simulink model "Breach_monitoring_subsystem"  (R2019b)
settings: Solver=VariableStepAuto  StartTime=0.0  StopTime=11.0  RelTol=1e-3
undefined symbols (not defined in the file or in its folder): nb_rooms, nb_step_to_fifteen_min, nb_step_to_one_h, nb_step_to_thirty_min
libraries: slstlib x6, dspstat3 x6
settings Model: Creator=pat  LastModifiedBy=pat

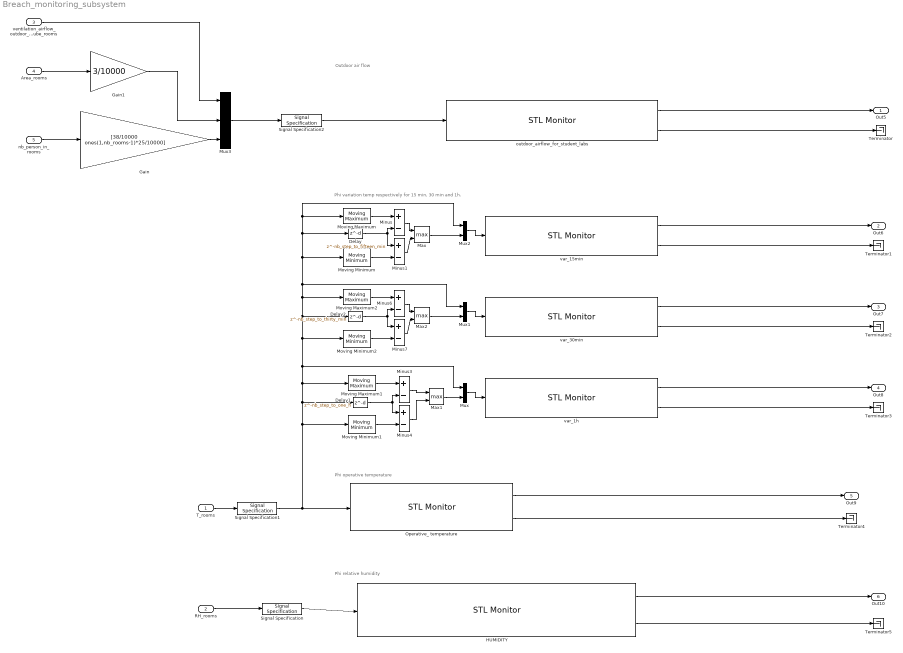
== system Breach_monitoring_subsystem ==
  note: Outdoor air flow
  note: Phi relative humidity
  note: Phi variation temp respectively for 15 min, 30 min and 1h.
  note: Phi operative temperature
  T_rooms : Inport  PortDimensions=nb_rooms
  RH_rooms : Inport  Port=2  PortDimensions=nb_rooms
  ventilation_airflow_outdoor_air_mcube_rooms : Inport  Port=3  PortDimensions=nb_rooms
  Area_rooms : Inport  Port=4  PortDimensions=nb_rooms
  nb_person_in_rooms : Inport  Port=5  OutDataTypeStr=double  PortDimensions=nb_rooms
  Delay : Delay  DelayLength=nb_step_to_fifteen_min  InitialCondition=0
  Delay1 : Delay  DelayLength=nb_step_to_one_h  InitialCondition=0
  Delay2 : Delay  DelayLength=nb_step_to_thirty_min  InitialCondition=0
  Gain : Gain  Gain=[38/10000 ones(1,nb_rooms-1)*25/10000]
  Gain1 : Gain  Gain=3/10000
  "HUMIDITY " : slstlib/STL Monitor  SignalNames=name_rh  STLString=formula_rh  MaxRob=1  RefreshRate=rate  rob_low_lim=inf  rob_up_lim=-inf  rob_diff_lim=-inf
      settings: SourceProductName=Breach Library
  Max : MinMax  Function=max  Inputs=2
  Max1 : MinMax  Function=max  Inputs=2
  Max2 : MinMax  Function=max  Inputs=2
  Minus{,1,3..4,6..7} (6 alike) : Sum  Inputs=+-
  Moving Maximum : dspstat3/Moving Maximum  SpecifyWindowLength=on  WindowLength=nb_step_to_fifteen_min  SimulateUsing=Code generation
      settings: SourceProductName=DSP System Toolbox  SourceProductBaseCode=DS
  Moving Maximum1 : dspstat3/Moving Maximum  SpecifyWindowLength=on  WindowLength=nb_step_to_one_h  SimulateUsing=Code generation
      settings: SourceProductName=DSP System Toolbox  SourceProductBaseCode=DS
  Moving Maximum2 : dspstat3/Moving Maximum  SpecifyWindowLength=on  WindowLength=nb_step_to_thirty_min  SimulateUsing=Code generation
      settings: SourceProductName=DSP System Toolbox  SourceProductBaseCode=DS
  Moving Minimum : dspstat3/Moving Minimum  SpecifyWindowLength=on  WindowLength=nb_step_to_fifteen_min  SimulateUsing=Code generation
      settings: SourceProductName=DSP System Toolbox  SourceProductBaseCode=DS
  Moving Minimum1 : dspstat3/Moving Minimum  SpecifyWindowLength=on  WindowLength=nb_step_to_one_h  SimulateUsing=Code generation
      settings: SourceProductName=DSP System Toolbox  SourceProductBaseCode=DS
  Moving Minimum2 : dspstat3/Moving Minimum  SpecifyWindowLength=on  WindowLength=nb_step_to_thirty_min  SimulateUsing=Code generation
      settings: SourceProductName=DSP System Toolbox  SourceProductBaseCode=DS
  Mux : Mux  Inputs=2
  Mux1 : Mux  Inputs=2
  Mux2 : Mux  Inputs=2
  Mux3 : Mux  Inputs=[nb_rooms nb_rooms nb_rooms]
  Operative_ temperature : slstlib/STL Monitor  SignalNames=name_op_temp  STLString=formula_op_temp  MaxRob=40  RefreshRate=rate  rob_low_lim=inf  rob_up_lim=-inf  rob_diff_lim=-inf
      settings: SourceProductName=Breach Library
  Signal Specification : SignalSpecification  OutMin=-0.25  OutMax=1.25  Dimensions=nb_rooms
  Signal Specification1 : SignalSpecification  OutMin=-100  OutMax=100  Dimensions=nb_rooms
  Signal Specification2 : SignalSpecification  OutMin=-10000  OutMax=10000  Dimensions=nb_rooms*3
  Terminator{,1..5} (6 alike) : Terminator
  outdoor_airflow_for_student_labs : slstlib/STL Monitor  SignalNames=name_out_airflow  STLString=formula_out_airflow  MaxRob=40  RefreshRate=rate  rob_low_lim=inf  rob_up_lim=-inf  rob_diff_lim=-inf
      settings: SourceProductName=Breach Library
  var_15min : slstlib/STL Monitor  SignalNames=name_variation  STLString=formula_fifteen_min_var  MaxRob=2  RefreshRate=rate  rob_low_lim=inf  rob_up_lim=-inf  rob_diff_lim=-inf
      settings: SourceProductName=Breach Library
  var_1h : slstlib/STL Monitor  SignalNames=name_variation  STLString=formula_one_h_var  MaxRob=2  RefreshRate=rate  rob_low_lim=inf  rob_up_lim=-inf  rob_diff_lim=-inf
      settings: SourceProductName=Breach Library
  var_30min : slstlib/STL Monitor  SignalNames=name_variation  STLString=formula_thirty_min_var  MaxRob=2  RefreshRate=rate  rob_low_lim=inf  rob_up_lim=-inf  rob_diff_lim=-inf
      settings: SourceProductName=Breach Library
  Out5 : Outport
  Out6 : Outport  Port=2
  Out7 : Outport  Port=3
  Out8 : Outport  Port=4
  Out9 : Outport  Port=5
  Out10 : Outport  Port=6
  wires:
  RH_rooms/1 -> Signal Specification/1
  Operative_ temperature/2 -> Terminator4/1
  Operative_ temperature/1 -> Out9/1
  Moving Maximum/1 -> Minus/1
  Delay/1 -> Minus1/1, Minus/2
  Moving Minimum/1 -> Minus1/2
  Minus/1 -> Max/1
  Minus1/1 -> Max/2
  Moving Minimum1/1 -> Minus4/2
  Minus3/1 -> Max1/1
  Delay1/1 -> Minus3/2, Minus4/1
  Minus4/1 -> Max1/2
  Moving Maximum1/1 -> Minus3/1
  Moving Minimum2/1 -> Minus7/2
  Minus6/1 -> Max2/1
  Delay2/1 -> Minus6/2, Minus7/1
  Minus7/1 -> Max2/2
  Moving Maximum2/1 -> Minus6/1
  Max/1 -> Mux2/2
  Max2/1 -> Mux1/2
  Max1/1 -> Mux/2
  ventilation_airflow_outdoor_air_mcube_rooms/1 -> Mux3/1
  outdoor_airflow_for_student_labs/2 -> Terminator/1
  var_15min/2 -> Terminator1/1
  var_30min/2 -> Terminator2/1
  var_1h/2 -> Terminator3/1
  "HUMIDITY "/2 -> Terminator5/1
  var_1h/1 -> Out8/1
  var_30min/1 -> Out7/1
  var_15min/1 -> Out6/1
  outdoor_airflow_for_student_labs/1 -> Out5/1
  Mux/1 -> var_1h/1
  Mux1/1 -> var_30min/1
  Mux2/1 -> var_15min/1
  T_rooms/1 -> Signal Specification1/1
  Mux3/1 -> Signal Specification2/1
  nb_person_in_rooms/1 -> Gain/1
  Area_rooms/1 -> Gain1/1
  Gain1/1 -> Mux3/2
  Gain/1 -> Mux3/3
  Signal Specification/1 -> "HUMIDITY "/1
  Signal Specification1/1 -> Delay1/1, Mux/1, Mux1/1, Delay/1, Mux2/1, Moving Maximum/1, Moving Minimum/1, Moving Maximum2/1, Delay2/1, Moving Minimum2/1, Moving Maximum1/1, Moving Minimum1/1, Operative_ temperature/1
  Signal Specification2/1 -> outdoor_airflow_for_student_labs/1
  "HUMIDITY "/1 -> Out10/1
